simulink model "LinearControl"  (R2024b)
settings: Solver=VariableStepAuto  StartTime=0.0  StopTime=T  RelTol=1e-3
InitFcn:
  | leminscate;
StopFcn:
  | plottingLinear;
values from neighbouring files (symbols this model uses):
  Ts = 0.01    [leminscate.m]
libraries: robotmobilelib x1
settings Model: Creator=salva  LastModifiedBy=salva

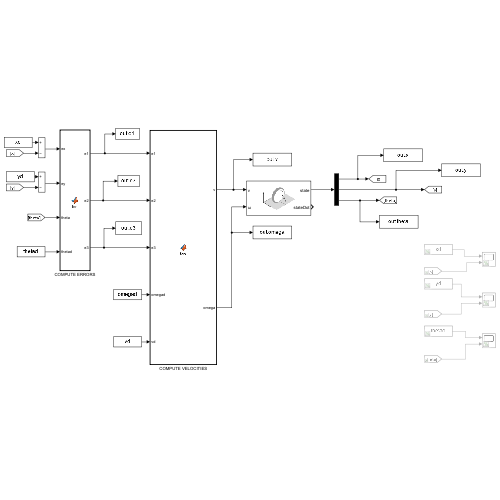
[thumbnail: Simulink's stored preview of the top-level diagram]
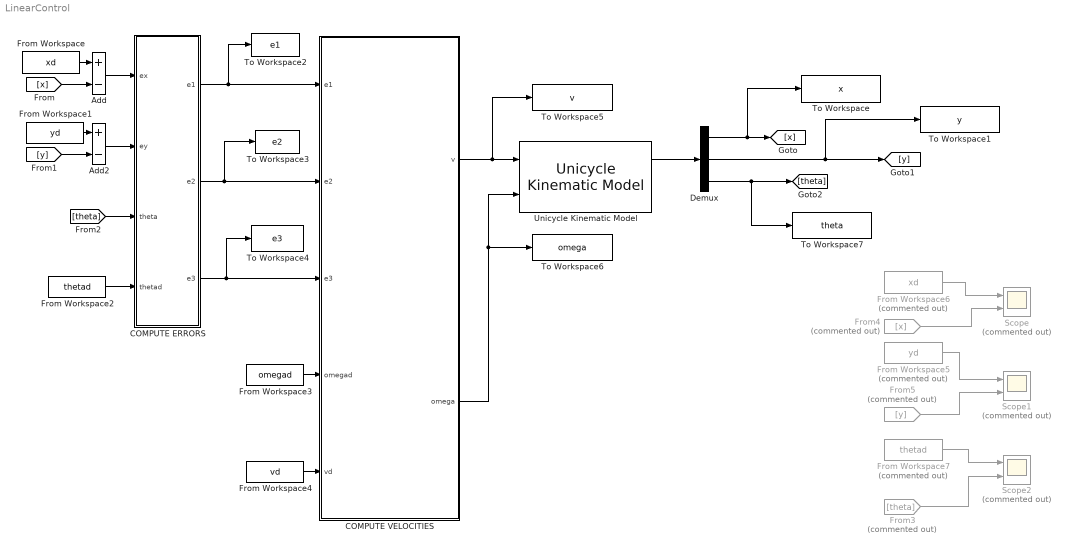
== system LinearControl ==
  Add : Sum  Inputs=+-
  Add2 : Sum  Inputs=+-
  COMPUTE ERRORS : MATLAB Function  TreatAsAtomicUnit=on
  COMPUTE VELOCITIES : MATLAB Function  TreatAsAtomicUnit=on
  Demux : Demux  Outputs=3
  From Workspace : FromWorkspace  VariableName=xd
  From Workspace1 : FromWorkspace  VariableName=yd
  From Workspace2 : FromWorkspace  VariableName=thetad
  From Workspace3 : FromWorkspace  VariableName=omegad
  From Workspace4 : FromWorkspace  VariableName=vd
  From Workspace5 : FromWorkspace  Commented=on  VariableName=yd
  From Workspace6 : FromWorkspace  Commented=on  VariableName=xd
  From Workspace7 : FromWorkspace  Commented=on  VariableName=thetad
  From3 : From  Commented=on  GotoTag=theta
  From4 : From  Commented=on  GotoTag=x
  From5 : From  Commented=on  GotoTag=y
  Scope : Scope  Commented=on  NumInputPorts=2
  Scope1 : Scope  Commented=on  NumInputPorts=2
  Scope2 : Scope  Commented=on  NumInputPorts=2
  To Workspace : ToWorkspace  VariableName=x  SaveFormat=Timeseries  SampleTime=Ts
  To Workspace1 : ToWorkspace  VariableName=y  SaveFormat=Timeseries  SampleTime=Ts
  To Workspace2 : ToWorkspace  VariableName=e1  SaveFormat=Timeseries  SampleTime=Ts
  To Workspace3 : ToWorkspace  VariableName=e2  SaveFormat=Timeseries  SampleTime=Ts
  To Workspace4 : ToWorkspace  VariableName=e3  SaveFormat=Timeseries  SampleTime=Ts
  To Workspace5 : ToWorkspace  VariableName=v  SaveFormat=Timeseries  SampleTime=Ts
  To Workspace6 : ToWorkspace  VariableName=omega  SaveFormat=Timeseries  SampleTime=Ts
  To Workspace7 : ToWorkspace  VariableName=theta  SaveFormat=Timeseries  SampleTime=-1
  Unicycle Kinematic Model : robotmobilelib/Unicycle Kinematic Model  VehicleInputs=Vehicle Speed & Heading Angular Velocity  WheelRadius=R  WheelSpeedRange=[-Inf,Inf]  InitialState=qi  SimulateUsing=Interpreted execution
  wires:
  Demux/1 -> To Workspace/1, [x]
  Unicycle Kinematic Model/1 -> Demux/1
  Demux/2 -> To Workspace1/1, [y]
  Demux/3 -> To Workspace7/1, [theta]
  From Workspace/1 -> Add/1
  [x] -> Add/2
  From Workspace1/1 -> Add2/1
  [y] -> Add2/2
  Add/1 -> COMPUTE ERRORS/1(ex)
  From Workspace2/1 -> COMPUTE ERRORS/4(thetad)
  [theta] -> COMPUTE ERRORS/3(theta)
  Add2/1 -> COMPUTE ERRORS/2(ey)
  COMPUTE ERRORS/1(e1) -> COMPUTE VELOCITIES/1(e1), To Workspace2/1
  COMPUTE ERRORS/2(e2) -> COMPUTE VELOCITIES/2(e2), To Workspace3/1
  COMPUTE ERRORS/3(e3) -> To Workspace4/1, COMPUTE VELOCITIES/3(e3)
  From Workspace3/1 -> COMPUTE VELOCITIES/4(omegad)
  From Workspace4/1 -> COMPUTE VELOCITIES/5(vd)
  COMPUTE VELOCITIES/1(v) -> To Workspace5/1, Unicycle Kinematic Model/1
  COMPUTE VELOCITIES/2(omega) -> To Workspace6/1, Unicycle Kinematic Model/2
  From Workspace6/1 -> Scope/1
  From4/1 -> Scope/2
  From5/1 -> Scope1/2
  From Workspace5/1 -> Scope1/1
  From Workspace7/1 -> Scope2/1
  From3/1 -> Scope2/2

== matlab function LinearControl/COMPUTE VELOCITIES ==
  data: e1 input; v output; e2 input; e3 input; omegad input; vd input; omega output
function [v,omega] = fcn(e1,e2,e3,omegad,vd)

    zita=0.7;
    a=90;
    k1=2*zita*a;
    k3=k1;
    
    k2=(a^2-omegad)/vd;
    
    %virtual inputs
    u1=-k1*e1;
    u2=-k2*e2-k3*e3;
    
    %actual outputs
    v=vd*cos(e3)-u1;
    omega=omegad-u2;

end

== matlab function LinearControl/COMPUTE ERRORS ==
  data: ex input; e1 output; ey input; theta input; e2 output; e3 output; thetad input
%Represent the errors in the current heading direction
function [e1,e2,e3] = fcn(ex,ey,theta,thetad)

    T=[cos(theta),sin(theta),0;
        -sin(theta),cos(theta),0;
        0,0,1];
    
    res=T*[ex;ey;thetad-theta];
    
    e1=res(1);
    e2=res(2);
    e3=res(3);

end
